simulink model "Cowley436HW2"  (R2022b)
settings: Solver=FixedStepAuto  StartTime=0.0  StopTime=50  FixedStep=0.1  RelTol=1e-3
values from neighbouring files (symbols this model uses):
  b = 0.25    [Cowley_436HW2.m]    (also in Cowley_MME436Lab3.m = 0.1; poleIdentification.m = 2*wn*zeta; tfCharacterisitcs.m = 2)
  br = 0.25    [Cowley_436HW2.m]
  F = 1    [Cowley_436HW2.m]
  J = 1    [Cowley_436HW2.m]    (also in Cowley_MME436Lab3.m = 0.01)
  k = 1    [Cowley_436HW2.m]
  kr = 0.5    [Cowley_436HW2.m]
  m = 0.5    [Cowley_436HW2.m]
  r = 0.4    [Cowley_436HW2.m]
settings Model: Creator=mattcowley  LastModifiedBy=mattcowley

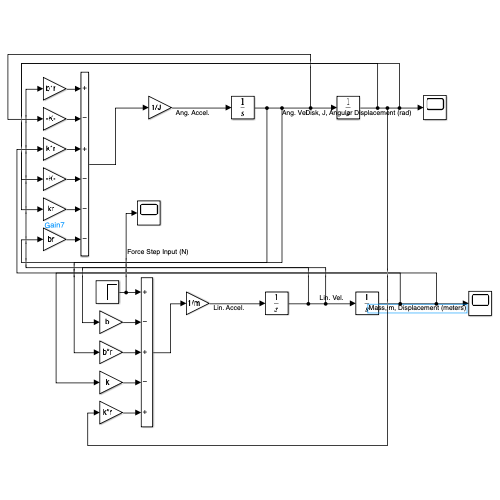
[thumbnail: Simulink's stored preview of the top-level diagram]
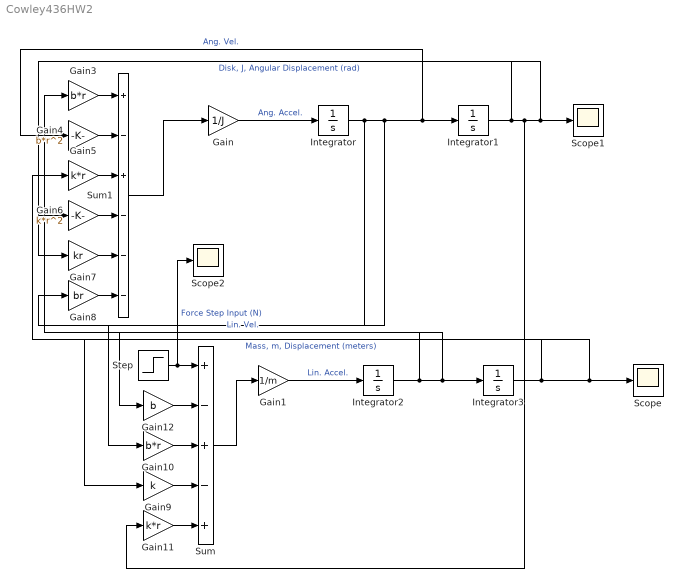
== system Cowley436HW2 ==
  Gain : Gain  Gain=1/J
  Gain1 : Gain  Gain=1/m
  Gain10 : Gain  Gain=b*r
  Gain11 : Gain  Gain=k*r
  Gain12 : Gain  Gain=b
  Gain3 : Gain  Gain=b*r
  Gain4 : Gain  Gain=b*r^2
  Gain5 : Gain  Gain=k*r
  Gain6 : Gain  Gain=k*r^2
  Gain7 : Gain  Gain=kr
  Gain8 : Gain  Gain=br
  Gain9 : Gain  Gain=k
  Integrator{,1..3} (4 alike) : Integrator
  Scope : Scope
  Scope1 : Scope
  Scope2 : Scope
  Step : Step  Time=0  Before=F  SampleTime=0
  Sum : Sum  Inputs=+-+-+
  Sum1 : Sum  Inputs=+-+---
  wires:
  Integrator/1 -> Gain10/1, Gain8/1, Gain4/1, Integrator1/1  "Ang. Vel."
  Gain/1 -> Integrator/1  "Ang. Accel."
  Integrator2/1 -> Gain12/1, Gain3/1, Integrator3/1  "Lin. Vel."
  Gain1/1 -> Integrator2/1  "Lin. Accel."
  Integrator3/1 -> Gain9/1, Gain5/1, Scope/1  "Mass, m, Displacement (meters)"
  Integrator1/1 -> Gain7/1, Gain11/1, Gain6/1, Scope1/1  "Disk, J, Angular Displacement (rad)"
  Sum/1 -> Gain1/1
  Sum1/1 -> Gain/1
  Gain8/1 -> Sum1/6
  Gain7/1 -> Sum1/5
  Gain6/1 -> Sum1/4
  Gain5/1 -> Sum1/3
  Gain4/1 -> Sum1/2
  Gain3/1 -> Sum1/1
  Step/1 -> Scope2/1, Sum/1  "Force Step Input (N)"
  Gain12/1 -> Sum/2
  Gain10/1 -> Sum/3
  Gain9/1 -> Sum/4
  Gain11/1 -> Sum/5
